simulink model "sldemo_bumpless_org"  (Simulink 10.0)
settings: Solver=ode45  StartTime=0.0  StopTime=600  MaxStep=0.1  RelTol=1e-5  EnableMultiTasking=on
libraries: simulink x4
settings Model: Creator=The MathWorks, Inc.  LastModifiedBy=bhisma
settings DataIOCC: LimitDataPoints=on
settings OptimizationCC: ExpressionDepthLimit=2147483647
settings DebuggingCC: UnderspecifiedInitializationDetection=Simplified  MergeDetectMultiDrivingBlocksExec=error  SolverPrmCheckMsg=warning  FcnCallInpInsideContextMsg=warning  StateNameClashWarn=warning
settings GRTTargetCC: GeneratePreprocessorConditionals=Disable all
settings ConfigComp: CovExternalEMLEnable=off

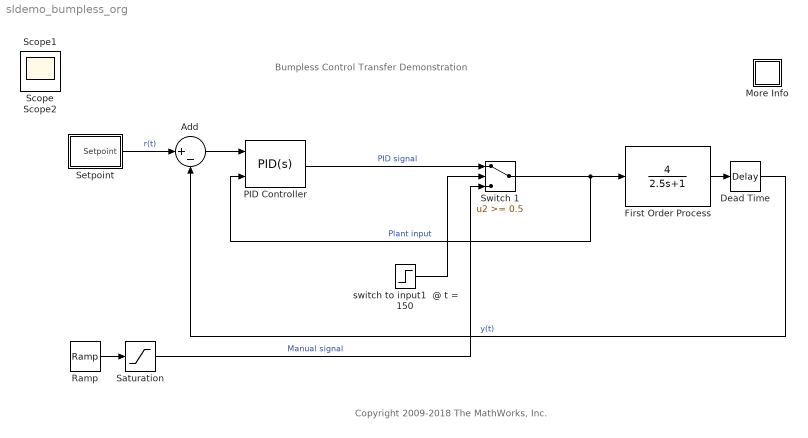
== system sldemo_bumpless_org ==
  note: Bumpless Control Transfer Demonstration
  note: Copyright 2009-2018 The MathWorks, Inc.
  Add : Sum  Inputs=|+-
  Dead Time : TransportDelay  BufferSize=2048
  First Order Process : TransferFcn  Numerator=4  Denominator=[2.5 1]
  More Info : Subsystem
      settings: OpenFcn=showdemo('sldemo_bumpless')
      mask Display: disp('?')
  PID Controller : simulink/Continuous/PID Controller  Controller=PID  Form=Parallel  TimeDomain=Continuous-time  SampleTime=-1  IntegratorMethod=Forward Euler  FilterMethod=Forward Euler  ControllerParametersSource=internal  P=0.32051437453006  I=0.13025295582387  D=0  UseFilter=on  N=100  TunerSelectOption=Transfer Function Based (PID Tuner App)  InitialConditionSource=internal  InitialConditionForIntegrator=0  InitialConditionForFilter=0  DifferentiatorICPrevScaledInput=0  ExternalReset=none  TrackingMode=on  Kt=1  LimitOutput=off  UpperSaturationLimit=inf  LowerSaturationLimit=-inf  LinearizeAsGain=off  AntiWindupMode=none  Kb=1  POutMin=[]  POutMax=[]  IOutMin=[]  IOutMax=[]  DOutMin=[]  DOutMax=[]  NOutMin=[]  NOutMax=[]  SumOutMin=[]  SumOutMax=[]  SaturationOutMin=[]  SaturationOutMax=[]  PParamMin=[]  PParamMax=[]  IParamMin=[]  IParamMax=[]  DParamMin=[]  DParamMax=[]  NParamMin=[]  NParamMax=[]  KbParamMin=[]  KbParamMax=[]  KtParamMin=[]  KtParamMax=[]  KbOutMin=[]  KbOutMax=[]  KtOutMin=[]  KtOutMax=[]  IntegratorOutMin=[]  IntegratorOutMax=[]  FilterOutMin=[]  FilterOutMax=[]  SumI1OutMin=[]  SumI1OutMax=[]  SumI2OutMin=[]  SumI2OutMax=[]  SumI3OutMin=[]  SumI3OutMax=[]  SumI4OutMin=[]  SumI4OutMax=[]  SumDOutMin=[]  SumDOutMax=[]  DifferentiatorOutMin=[]  DifferentiatorOutMax=[]  FilterDiffOutCoefMin=[]  FilterDiffOutCoefMax=[]  ReciprocalOutMin=[]  ReciprocalOutMax=[]  SumDenOutMin=[]  SumDenOutMax=[]  SumNumOutMin=[]  SumNumOutMax=[]  DivideOutMin=[]  DivideOutMax=[]  IntegratorContinuousStateAttributes=''  IntegratorStateMustResolveToSignalObject=off  IntegratorRTWStateStorageClass=Auto  FilterContinuousStateAttributes=''  FilterStateMustResolveToSignalObject=off  FilterRTWStateStorageClass=Auto  ParallelPVariant=InternalParameters  IdealPVariant=Disabled  IVariant=InternalParameters  DVariant=InternalParameters  IntegratorVariant=Continuous  SatVariant=Disabled  AWVariant=Passthrough  PCopyVariant=Disabled  TRVariant=Enabled  FdbkBlocksVariant=Forward  IdealPFdbkVariant=Disabled  SatFdbkVariant=Disabled  DerivativeFilterVariant=ContFilter  NVariant=InternalParameters  NCopyVariant=Disabled  FilterICVariant=InternalICsFilter  IntegratorICVariant=InternalICs  ExternalResetVariant=Disabled  TRSumVariant=TrackingMode  SumFdbkVariant=Disabled  SumVariant=Sum_PID
  Ramp : simulink/Sources/Ramp  slope=0.1  start=0  InitialOutput=0
  Saturation : Saturate  UpperLimit=10  LowerLimit=-10
  Setpoint : Subsystem
  Switch 1 : Switch  Threshold=0.5
  switch to input1  @ t = 150 : Step  Time=150  SampleTime=0
  Scope : Scope
  Scope1 : Scope
  Scope2 : Scope
  wires:
  Add/1 -> PID Controller/1
  Dead Time/1 -> Add/2  "y(t)"
  Switch 1/1 -> First Order Process/1, PID Controller/2  "Plant input"
  PID Controller/1 -> Switch 1/1  "PID signal"
  Saturation/1 -> Switch 1/3  "Manual signal"
  Setpoint/1(Setpoint) -> Add/1  "r(t)"
  First Order Process/1 -> Dead Time/1
  switch to input1  @ t = 150/1 -> Switch 1/2
  Ramp/1 -> Saturation/1

== system sldemo_bumpless_org/More Info ==

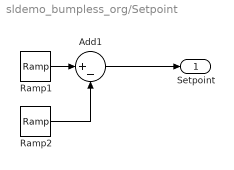
== system sldemo_bumpless_org/Setpoint ==
  Add1 : Sum  Inputs=|+-
  Ramp1 : simulink/Sources/Ramp  slope=-0.125  start=320  InitialOutput=40
  Ramp2 : simulink/Sources/Ramp  slope=-0.125  start=480  InitialOutput=0
  Setpoint : Outport  VectorParamsAs1DForOutWhenUnconnected=off
  wires:
  Ramp2/1 -> Add1/2
  Ramp1/1 -> Add1/1
  Add1/1 -> Setpoint/1
